simulink model "problematique2"  (Simulink 10.2)
settings: Solver=ode4  StartTime=0.0  StopTime=SIMULPARAM.T_end  FixedStep=SIMULPARAM.Ts  RelTol=1e-3  EnableMultiTasking=on
undefined symbols (not defined in the file): BAT, C_speed, CHAS, Chopper, CYCL, d_current_control, DCBUSCONTROL, dCURRENTCONTROL, ENV, Flux_control, FLUXCONTROL, FLUXSTRATEGY, IM, L, q_current_control, qCURRENTCONTROL, SC, SCCURRENTCONTROL, STRATEGY, TRANS
libraries: simulink x3, cstblocks x1
settings Model: Creator=Huy  LastModifiedBy=mikesimard
settings SolverCC: AlgebraicLoopSolver=LineSearch  AutoInsertRateTranBlk=on
settings DataIOCC: SaveOutput=off  SignalLogging=off  SaveTime=off
settings OptimizationCC: ExpressionDepthLimit=2147483647
settings DebuggingCC: AlgebraicLoopMsg=none  SaveWithDisabledLinksMsg=none  MaxConsecutiveZCsMsg=none  SolverPrmCheckMsg=warning  ModelReferenceDataLoggingMessage=none  ModelReferenceExtraNoncontSigs=none  StateNameClashWarn=warning

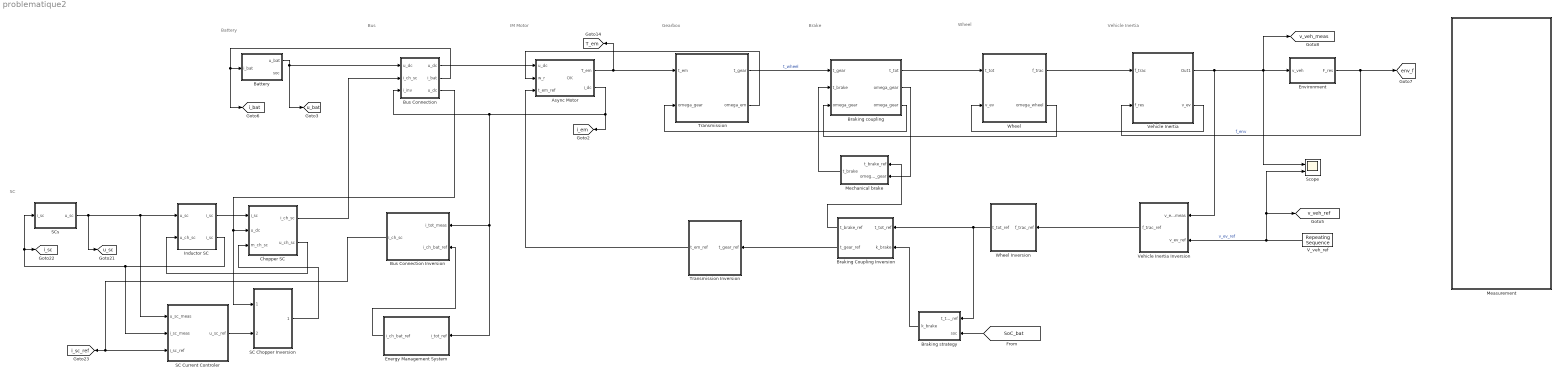
== system problematique2 ==
  note: Battery
  note: Bus
  note: IM Motor
  note: Gearbox
  note: Brake
  note: Wheel
  note: Vehicle Inertia
  note: SC
  note: OK
  Async Motor : Subsystem
  Battery : Subsystem  AncestorBlock=simulink/REM/SE
      mask Display:
      | plot(0,0,100,100, 1.2*[50,57.68,60.77,63.08,64.97,66.58,68,69.26,70.4, 	71.42,72.36,78.28,80,78.28,72.36,71.42,70.4, 	69.26,68,66.58,64.97,63.08,60.77,57.68,50,42.32, 	39.23,36.92,35.03,33.42,32,30.74,29.6,28.58, 	27.64,21.72,20,21.72,27.64,28.58,29.6,30.74,32, 	33.42,35.03,36.92,39.23,42.32,50]-10, 1.2*[20,21,22,23,24,25,26,27,28,29,30,40,50,60,70,71,72, 	73,74,75,76,77,78,79,80,79,78,77,76,75,74,73,72, 	71,70,60,50,40,30,29,28,27,26,25,24,23,22,21,20]-10)
      | disp('ES')
  Braking Coupling Inversion : Subsystem  AncestorBlock=simulink/SMC/Bloc de répartition
      mask Display: plot(0,0,100,100,[20,40,100,80,20],[75,20,20,75,75], [0,20,80,60,0],[85,30,30,85,85])
  Braking coupling : Subsystem  mask(CM){}
      mask Display: plot(0,0,100,100,[35,35,95,95,35],[65,10,10,65,65], [5,5,65,65,5],[90,35,35,90,90])
  Braking strategy : Subsystem  AncestorBlock=simulink/SMC/Inversion EC avec mesure
      mask Display: plot(0,0,100,100,[10,30,90,70,10],[90,10,10,90,90])
  Bus Connection : Subsystem  mask(CM){}
      mask Display: plot(0,0,100,100,[35,35,95,95,35],[65,10,10,65,65], [5,5,65,65,5],[90,35,35,90,90])
  Bus Connection Inversion : Subsystem  AncestorBlock=simulink/SMC/Bloc de répartition
      mask Display: plot(0,0,100,100,[20,40,100,80,20],[75,20,20,75,75], [0,20,80,60,0],[85,30,30,85,85])
  Chopper SC : Subsystem  AncestorBlock=simulink/REM/EC Elec  mask(Hacheur){}
      mask Display: plot(0,0,100,100,[10,10,90,90,10],[90,10,10,90,90])
  Energy Management System : Subsystem  AncestorBlock=simulink/SMC/Inversion EC avec mesure
      mask Display: plot(0,0,100,100,[10,30,90,70,10],[90,10,10,90,90])
  Environment : Subsystem  AncestorBlock=simulink/REM/SE
      mask Display:
      | plot(0,0,100,100, 1.2*[50,57.68,60.77,63.08,64.97,66.58,68,69.26,70.4, 	71.42,72.36,78.28,80,78.28,72.36,71.42,70.4, 	69.26,68,66.58,64.97,63.08,60.77,57.68,50,42.32, 	39.23,36.92,35.03,33.42,32,30.74,29.6,28.58, 	27.64,21.72,20,21.72,27.64,28.58,29.6,30.74,32, 	33.42,35.03,36.92,39.23,42.32,50]-10, 1.2*[20,21,22,23,24,25,26,27,28,29,30,40,50,60,70,71,72, 	73,74,75,76,77,78,79,80,79,78,77,76,75,74,73,72, 	71,70,60,50,40,30,29,28,27,26,25,24,23,22,21,20]-10)
      | disp('MS')
  Inductor SC : Subsystem  AncestorBlock=simulink/REM/EA  mask(CM){}
      mask Display: plot(0,0,100,100,[10,10,90,90,10],[90,10,10,90,90], [10,90],[10,90])
  Measurement : Subsystem
  Mechanical brake : Subsystem  AncestorBlock=simulink/REM/SE
      mask Display:
      | plot(0,0,100,100, 1.2*[50,57.68,60.77,63.08,64.97,66.58,68,69.26,70.4, 	71.42,72.36,78.28,80,78.28,72.36,71.42,70.4, 	69.26,68,66.58,64.97,63.08,60.77,57.68,50,42.32, 	39.23,36.92,35.03,33.42,32,30.74,29.6,28.58, 	27.64,21.72,20,21.72,27.64,28.58,29.6,30.74,32, 	33.42,35.03,36.92,39.23,42.32,50]-10, 1.2*[20,21,22,23,24,25,26,27,28,29,30,40,50,60,70,71,72, 	73,74,75,76,77,78,79,80,79,78,77,76,75,74,73,72, 	71,70,60,50,40,30,29,28,27,26,25,24,23,22,21,20]-10)
      | disp('MS')
  SC Chopper Inversion : Subsystem
      mask Display: plot(0,0,100,100,[10,30,90,70,10],[90,10,10,90,90])
  SC Current Controler : Subsystem
      mask Display: plot(0,0,100,100, [10,30,90,70,10,90],[90,10,10,90,90,10])
  SCs : Subsystem  AncestorBlock=simulink/REM/SE
      mask Display:
      | plot(0,0,100,100, 1.2*[50,57.68,60.77,63.08,64.97,66.58,68,69.26,70.4, 	71.42,72.36,78.28,80,78.28,72.36,71.42,70.4, 	69.26,68,66.58,64.97,63.08,60.77,57.68,50,42.32, 	39.23,36.92,35.03,33.42,32,30.74,29.6,28.58, 	27.64,21.72,20,21.72,27.64,28.58,29.6,30.74,32, 	33.42,35.03,36.92,39.23,42.32,50]-10, 1.2*[20,21,22,23,24,25,26,27,28,29,30,40,50,60,70,71,72, 	73,74,75,76,77,78,79,80,79,78,77,76,75,74,73,72, 	71,70,60,50,40,30,29,28,27,26,25,24,23,22,21,20]-10)
      | disp('ES')
  Scope : Scope  NumInputPorts=2
  Transmission : Subsystem  AncestorBlock=simulink/REM/EA  mask(CM){}
      mask Display: plot(0,0,100,100,[10,10,90,90,10],[90,10,10,90,90])
  Transmission Inversion : Subsystem  AncestorBlock=simulink/SMC/Inversion EC avec mesure
      mask Display: plot(0,0,100,100,[10,30,90,70,10],[90,10,10,90,90])
  V_veh_ref : simulink/Sources/Repeating Sequence  rep_seq_t=CYCL.time  rep_seq_y=CYCL.velocity/1.25
  Vehicle Inertia : Subsystem  AncestorBlock=simulink/REM/EA  mask(CM){}
      mask Display: plot(0,0,100,100,[10,10,90,90,10],[90,10,10,90,90], [10,90],[10,90])
  Vehicle Inertia Inversion : Subsystem  AncestorBlock=simulink/SMC/Asservissement Correcteur IP
      mask Display: plot(0,0,100,100, [10,30,90,70,10,90],[90,10,10,90,90,10])
  Wheel : Subsystem  AncestorBlock=simulink/REM/EA  mask(CM){}
      mask Display: plot(0,0,100,100,[10,10,90,90,10],[90,10,10,90,90])
  Wheel Inversion : Subsystem  AncestorBlock=simulink/SMC/Inversion EC avec mesure
      mask Display: plot(0,0,100,100,[10,30,90,70,10],[90,10,10,90,90])
  tag scope: T_em=global, env_f=global, i_bat=global, i_em=global, i_sc=global, i_sc_ref=global, u_bat=global, u_sc=global, v_veh_meas=global, v_veh_ref=global
  wires:
  Vehicle Inertia/1(Out1) -> Environment/1(v_veh), Scope/1, [v_veh_meas], Vehicle Inertia Inversion/1(v_ev_meas)
  Wheel/1(f_trac) -> Vehicle Inertia/1(f_trac)
  Environment/1(F_res) -> [env_f], Vehicle Inertia/2(f_res)  "f_env"
  Vehicle Inertia/2(v_ev) -> Wheel/2(v_ev)
  V_veh_ref/1 -> Scope/2, [v_veh_ref], Vehicle Inertia Inversion/2(v_ev_ref)  "v_ev_ref"
  Vehicle Inertia Inversion/1(f_trac_ref) -> Wheel Inversion/1(f_trac_ref)
  Transmission/1(t_gear) -> Braking coupling/1(t_gear)  "t_wheel"
  Mechanical brake/1(t_brake) -> Braking coupling/2(t_brake)
  Braking coupling/2(omega_gear) -> Mechanical brake/2(omega_gear)
  Braking Coupling Inversion/2(t_gear_ref) -> Transmission Inversion/1(t_gear_ref)
  Wheel Inversion/1(t_tot_ref) -> Braking strategy/1(t_tot_ref), Braking Coupling Inversion/1(t_tot_ref)
  Braking Coupling Inversion/1(t_brake_ref) -> Mechanical brake/1(t_brake_ref)
  Braking coupling/1(t_tot) -> Wheel/1(t_tot)
  Wheel/2(omega_wheel) -> Braking coupling/3("omega_gear  ")
  Braking coupling/3("omega_gear ") -> Transmission/2(omega_gear)
  Braking strategy/1(k_brake) -> Braking Coupling Inversion/2(k_brake)
  [SoC_bat] -> Braking strategy/2(soc)
  Async Motor/1(T_em) -> Transmission/1(t_em), [T_em]
  Chopper SC/2(u_ch_sc) -> Inductor SC/2(u_ch_sc)
  Inductor SC/1(i_sc) -> Chopper SC/1(i_sc)
  Async Motor/2(i_dc) -> Bus Connection/3(i_inv), Bus Connection Inversion/1(i_tot_meas), Energy Management System/1(i_tot_ref), [i_em]
  Energy Management System/1(i_ch_bat_ref) -> Bus Connection Inversion/2(i_ch_bat_ref)
  SCs/1(u_sc) -> [u_sc], SC Current Controler/1(u_sc_meas), Inductor SC/1(u_sc)
  SC Chopper Inversion/1(m_ch_sc) -> Chopper SC/3(m_ch_sc)
  SC Current Controler/1(u_sc_ref) -> SC Chopper Inversion/2(u_sc_ref)
  Inductor SC/2("i_sc ") -> SC Current Controler/2(i_sc_meas), SCs/1(i_sc), [i_sc]
  Bus Connection Inversion/1(i_ch_sc) -> [i_sc_ref], SC Current Controler/3(i_sc_ref)
  Battery/1(u_bat) -> [u_bat], Bus Connection/1(" u_dc ")
  Bus Connection/3("u_dc ") -> Chopper SC/2(u_dc), SC Chopper Inversion/1(u_dc_meas)
  Transmission/2(omega_em) -> Async Motor/2(w_r)
  Bus Connection/2(i_bat) -> [i_bat], Battery/1(i_bat)
  Bus Connection/1(u_dc) -> Async Motor/1(u_dc)
  Transmission Inversion/1(t_em_ref) -> Async Motor/3(t_em_ref)
  Chopper SC/1(i_ch_sc) -> Bus Connection/2(i_ch_sc)

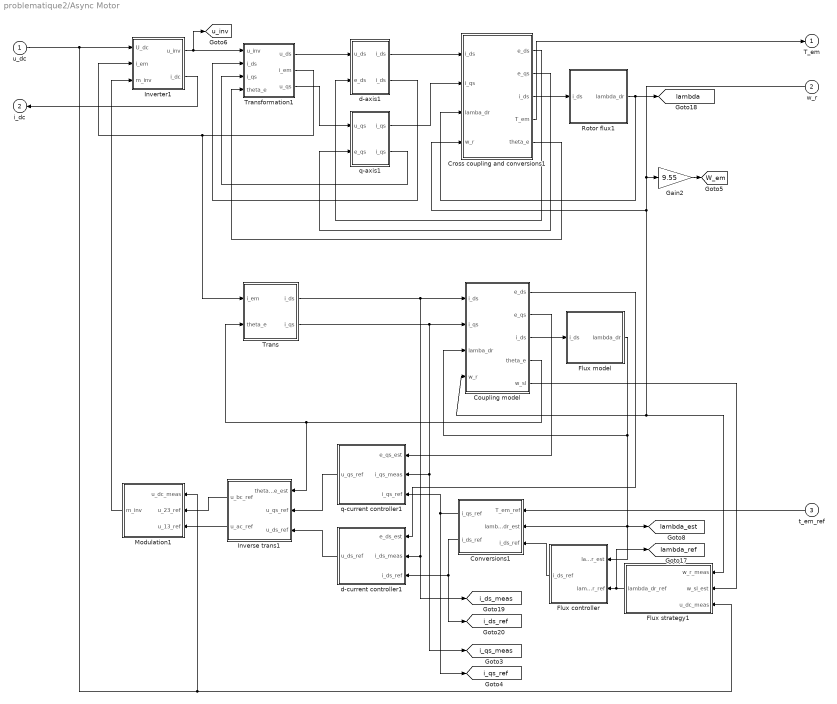
== system problematique2/Async Motor ==
  u_dc : Inport
  w_r : Inport  Port=2
  t_em_ref : Inport  Port=3
  Conversions1 : Subsystem  AncestorBlock=simulink/SMC/Bloc de répartition
      mask Display: plot(0,0,100,100,[20,40,100,80,20],[75,20,20,75,75], [0,20,80,60,0],[85,30,30,85,85])
  Coupling model : Subsystem  AncestorBlock=simulink/REM/EC EM
      mask Display: plot(0,0,100,100, [50,57.68,60.77,63.08,64.97,66.58,68,69.26,70.4, 	71.42,72.36,78.28,80,78.28,72.36,71.42,70.4, 	69.26,68,66.58,64.97,63.08,60.77,57.68,50,42.32, 	39.23,36.92,35.03,33.42,32,30.74,29.6,28.58, 	27.64,21.72,20,21.72,27.64,28.58,29.6,30.74,32, 	33.42,35.03,36.92,39.23,42.32,50], [20,21,22,23,24,25,26,27,28,29,30,40,50,60,70,71,72, 	73,74,75,76,77,78,79,80,79,78,77,76,75,74,73,72, 	71,70,60,50,40,30,29,28,27,26,25,24,23,22,21,20]-15,  [50,57.68,60.77,63.08,64.97,66.58,68,69.26,70.4, 	71.42,72.36,78.28,80,78.28,72.36,71.42,70.4, 	69.26,68,66.58,64.97,63.08,60.77,57.68,50,42.32, 	39.23,36.92,35.03,33.42,32,30.74,29.6,28.58, 	27.64,21.72,20,21.72,27.64,28.58,29.6,30.74,32, 	33.42,35.03,36.92,39.23,42.32,50], [20,21,22,23,24,25,26,27,28,29,30,40,50,60,70,71,72, 	73,74,75,76,77,78,79,80,79,78,77,76,75,74,73,72, 	71,70,60,50,40,30,29,28,27,26,25,24,23,22,21,20]+15)
  Cross coupling and conversions1 : Subsystem  mask(CM){}
      mask Display: plot(0,0,100,100, [50,57.68,60.77,63.08,64.97,66.58,68,69.26,70.4, 	71.42,72.36,78.28,80,78.28,72.36,71.42,70.4, 	69.26,68,66.58,64.97,63.08,60.77,57.68,50,42.32, 	39.23,36.92,35.03,33.42,32,30.74,29.6,28.58, 	27.64,21.72,20,21.72,27.64,28.58,29.6,30.74,32, 	33.42,35.03,36.92,39.23,42.32,50], [20,21,22,23,24,25,26,27,28,29,30,40,50,60,70,71,72, 	73,74,75,76,77,78,79,80,79,78,77,76,75,74,73,72, 	71,70,60,50,40,30,29,28,27,26,25,24,23,22,21,20]-15,  [50,57.68,60.77,63.08,64.97,66.58,68,69.26,70.4, 	71.42,72.36,78.28,80,78.28,72.36,71.42,70.4, 	69.26,68,66.58,64.97,63.08,60.77,57.68,50,42.32, 	39.23,36.92,35.03,33.42,32,30.74,29.6,28.58, 	27.64,21.72,20,21.72,27.64,28.58,29.6,30.74,32, 	33.42,35.03,36.92,39.23,42.32,50], [20,21,22,23,24,25,26,27,28,29,30,40,50,60,70,71,72, 	73,74,75,76,77,78,79,80,79,78,77,76,75,74,73,72, 	71,70,60,50,40,30,29,28,27,26,25,24,23,22,21,20]+15)
  Flux controller : Subsystem  AncestorBlock=simulink/SMC/Asservissement Correcteur IP
      mask Display: plot(0,0,100,100, [10,30,90,70,10,90],[90,10,10,90,90,10])
  Flux model : Subsystem  AncestorBlock=simulink/REM/EA  mask(CM){}
      mask Display: plot(0,0,100,100,[10,10,90,90,10],[90,10,10,90,90], [10,90],[10,90])
  Flux strategy1 : Subsystem  AncestorBlock=simulink/SMC/Inversion EC avec mesure
      mask Display: plot(0,0,100,100,[10,30,90,70,10],[90,10,10,90,90])
  Gain2 : Gain  Gain=9.55
  Inverse trans1 : Subsystem  AncestorBlock=simulink/SMC/Bloc de répartition
      mask Display: plot(0,0,100,100,[20,40,100,80,20],[75,20,20,75,75], [0,20,80,60,0],[85,30,30,85,85])
  Inverter1 : Subsystem  AncestorBlock=simulink/REM/EC Elec  mask(Hacheur){}
      mask Display: plot(0,0,100,100,[10,10,90,90,10],[90,10,10,90,90])
  Modulation1 : Subsystem  AncestorBlock=simulink/SMC/Bloc de répartition
      mask Display: plot(0,0,100,100,[10,30,90,70,10],[90,10,10,90,90])
  Rotor flux1 : Subsystem  AncestorBlock=simulink/REM/EA  mask(CM){}
      mask Display: plot(0,0,100,100,[10,10,90,90,10],[90,10,10,90,90], [10,90],[10,90])
  Trans : Subsystem  mask(CM){}
      mask Display: plot(0,0,100,100,[35,35,95,95,35],[65,10,10,65,65], [5,5,65,65,5],[90,35,35,90,90])
  Transformation1 : Subsystem  mask(CM){}
      mask Display: plot(0,0,100,100,[35,35,95,95,35],[65,10,10,65,65], [5,5,65,65,5],[90,35,35,90,90])
  d-axis1 : Subsystem  AncestorBlock=simulink/REM/EA  mask(CM){}
      mask Display: plot(0,0,100,100,[10,10,90,90,10],[90,10,10,90,90], [10,90],[10,90])
  d-current controller1 : Subsystem  AncestorBlock=simulink/SMC/Asservissement Correcteur IP
      mask Display: plot(0,0,100,100, [10,30,90,70,10,90],[90,10,10,90,90,10])
  q-axis1 : Subsystem  AncestorBlock=simulink/REM/EA  mask(CM){}
      mask Display: plot(0,0,100,100,[10,10,90,90,10],[90,10,10,90,90], [10,90],[10,90])
  q-current controller1 : Subsystem  AncestorBlock=simulink/SMC/Asservissement Correcteur IP
      mask Display: plot(0,0,100,100, [10,30,90,70,10,90],[90,10,10,90,90,10])
  T_em : Outport
  i_dc : Outport  Port=2
  tag scope: W_em=global, i_ds_meas=global, i_ds_ref=global, i_qs_meas=global, i_qs_ref=global, lambda=global, lambda_est=global, lambda_ref=global, u_inv=global
  wires:
  Flux controller/1(i_ds_ref) -> Conversions1/3(i_ds_ref)
  Transformation1/1(u_ds) -> d-axis1/1(u_ds)
  Conversions1/2("i_ds_ref  ") -> d-current controller1/3(i_ds_ref), [i_ds_ref]
  d-axis1/1(i_ds) -> Cross coupling and conversions1/1(i_ds)
  q-axis1/2("i_qs ") -> Transformation1/3(i_qs)
  q-axis1/1(i_qs) -> Cross coupling and conversions1/2(i_qs)
  d-axis1/2("i_ds ") -> Transformation1/2(i_ds)
  Inverse trans1/1(u_bc_ref) -> Modulation1/2(u_23_ref)
  w_r/1 -> Flux strategy1/1(w_r_meas), Coupling model/4(w_r), Cross coupling and conversions1/4(w_r), Gain2/1
  q-current controller1/1(u_qs_ref) -> Inverse trans1/2(u_qs_ref)
  Rotor flux1/1(lambda_dr) -> Cross coupling and conversions1/3(lamba_dr), [lambda]
  Cross coupling and conversions1/4(T_em) -> T_em/1
  u_dc/1 -> Inverter1/1(U_dc), Modulation1/1(u_dc_meas), Flux strategy1/3(u_dc_meas)
  t_em_ref/1 -> Conversions1/1(T_em_ref)
  Inverter1/1(u_inv) -> [u_inv], Transformation1/1(u_inv)
  Coupling model/3("i_ds ") -> Flux model/1(i_ds)
  Gain2/1 -> [W_em]
  Coupling model/4(theta_e) -> Trans/2(theta_e), Inverse trans1/1(theta_e_est)
  Cross coupling and conversions1/3("i_ds ") -> Rotor flux1/1(i_ds)
  Conversions1/1(i_qs_ref) -> [i_qs_ref], q-current controller1/3(i_qs_ref)
  Transformation1/3(u_qs) -> q-axis1/1(u_qs)
  Transformation1/2(i_em) -> Inverter1/2(i_em), Trans/1(i_em)
  Coupling model/2(e_qs) -> q-current controller1/1(e_qs_est)
  Flux strategy1/1(lambda_dr_ref) -> [lambda_ref], Flux controller/2(lambda_dr_ref)
  Trans/1(i_ds) -> Coupling model/1(i_ds), [i_ds_meas], d-current controller1/2(i_ds_meas)
  d-current controller1/1(u_ds_ref) -> Inverse trans1/3(u_ds_ref)
  Cross coupling and conversions1/1(e_ds) -> d-axis1/2(e_ds)
  Coupling model/5(w_sl) -> Flux strategy1/2(w_sl_est)
  Modulation1/1(m_inv) -> Inverter1/3(m_inv)
  Trans/2(i_qs) -> Coupling model/2(i_qs), [i_qs_meas], q-current controller1/2(i_qs_meas)
  Cross coupling and conversions1/2(e_qs) -> q-axis1/2(e_qs)
  Coupling model/1(e_ds) -> d-current controller1/1(e_ds_est)
  Flux model/1(lambda_dr) -> Flux controller/1(lambda_dr_est), [lambda_est], Conversions1/2(lambda_dr_est), Coupling model/3(lamba_dr)
  Cross coupling and conversions1/5(theta_e) -> Transformation1/4(theta_e)
  Inverse trans1/2(u_ac_ref) -> Modulation1/3(u_13_ref)
  Inverter1/2(i_dc) -> i_dc/1

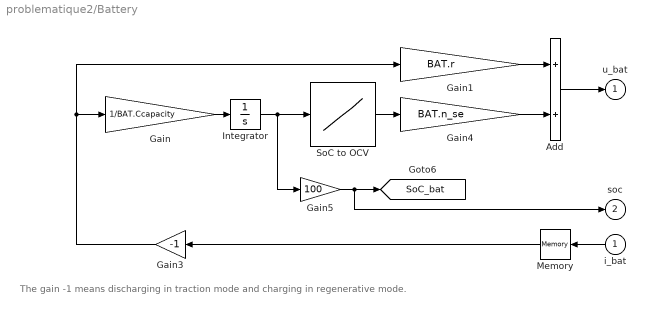
== system problematique2/Battery ==
  note: The gain -1 means discharging in traction mode and charging in regenerative mode.
  i_bat : Inport
  Add : Sum
  Gain : Gain  Gain=1/BAT.Ccapacity
  Gain1 : Gain  Gain=BAT.r
  Gain3 : Gain  Gain=-1
  Gain4 : Gain  Gain=BAT.n_se
  Gain5 : Gain  Gain=100
  Integrator : Integrator  InitialCondition=1
  Memory : Memory
  SoC to OCV : Lookup_n-D  NumberOfTableDimensions=1  BreakpointsForDimension1=0.2:0.1:1  Table=11.4:(12-11.4)/((1-0.2)/0.1):12  RndMeth=Simplest  InputSameDT=on
  u_bat : Outport  InitialOutput=0
  soc : Outport  Port=2  InitialOutput=0
  tag scope: SoC_bat=global
  wires:
  Gain5/1 -> soc/1, [SoC_bat]
  Memory/1 -> Gain3/1
  i_bat/1 -> Memory/1
  Gain/1 -> Integrator/1
  Gain3/1 -> Gain1/1, Gain/1
  SoC to OCV/1 -> Gain4/1
  Integrator/1 -> SoC to OCV/1, Gain5/1
  Gain1/1 -> Add/1
  Add/1 -> u_bat/1
  Gain4/1 -> Add/2

== system problematique2/Braking Coupling Inversion ==
  t_tot_ref : Inport
  k_brake : Inport  Port=2
  Abs : Abs
  Constant : Constant
  Product : Product  RndMeth=Zero
  Product1 : Product  RndMeth=Zero
  Sum : Sum  Inputs=+-
  t_brake_ref : Outport  InitialOutput=0  VectorParamsAs1DForOutWhenUnconnected=off
  t_gear_ref : Outport  Port=2  InitialOutput=0  VectorParamsAs1DForOutWhenUnconnected=off
  wires:
  Product1/1 -> t_gear_ref/1
  Sum/1 -> Product/2
  t_tot_ref/1 -> Product1/1, Product/1
  k_brake/1 -> Product1/2, Sum/2
  Constant/1 -> Sum/1
  Product/1 -> Abs/1
  Abs/1 -> t_brake_ref/1

== system problematique2/Braking coupling ==
  t_gear : Inport
  t_brake : Inport  Port=2
  "omega_gear  " : Inport  Port=3
  Sum : Sum  Inputs=|+-
  t_tot : Outport  InitialOutput=0  VectorParamsAs1DForOutWhenUnconnected=off
  omega_gear : Outport  Port=2  InitialOutput=0  VectorParamsAs1DForOutWhenUnconnected=off
  "omega_gear " : Outport  Port=3  InitialOutput=0  VectorParamsAs1DForOutWhenUnconnected=off
  wires:
  t_gear/1 -> Sum/1
  t_brake/1 -> Sum/2
  Sum/1 -> t_tot/1
  "omega_gear  "/1 -> omega_gear/1, "omega_gear "/1

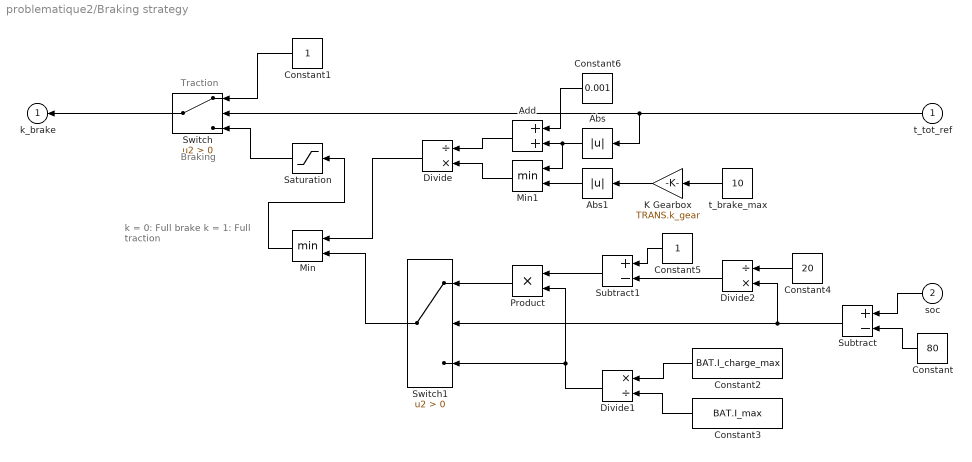
== system problematique2/Braking strategy ==
  note: k = 0: Full brake
      | k = 1: Full traction
  note: Traction
  note: Braking
  t_tot_ref : Inport
  soc : Inport  Port=2
  Abs : Abs
  Abs1 : Abs
  Add : Sum
  Constant : Constant  Value=80
  Constant1 : Constant
  Constant2 : Constant  Value=BAT.I_charge_max
  Constant3 : Constant  Value=BAT.I_max
  Constant4 : Constant  Value=20
  Constant5 : Constant
  Constant6 : Constant  Value=0.001
  Divide : Product  Inputs=/*
  Divide1 : Product  Inputs=*/
  Divide2 : Product  Inputs=/*
  K Gearbox : Gain  Gain=TRANS.k_gear
  Min : MinMax  Inputs=2
  Min1 : MinMax  Inputs=2
  Product : Product
  Saturation : Saturate  UpperLimit=1  LowerLimit=0
  Subtract : Sum  Inputs=+-
  Subtract1 : Sum  Inputs=+-
  Switch : Switch  Criteria=u2 > Threshold
  Switch1 : Switch  Criteria=u2 > Threshold
  t_brake_max : Constant  Value=10
  k_brake : Outport  InitialOutput=0  VectorParamsAs1DForOutWhenUnconnected=off
  wires:
  t_tot_ref/1 -> Abs/1, Switch/2
  Abs/1 -> Add/2, Min1/1
  Abs1/1 -> Min1/2
  Min1/1 -> Divide/2
  Constant/1 -> Subtract/2
  soc/1 -> Subtract/1
  Subtract/1 -> Divide2/2, Switch1/2
  Constant2/1 -> Divide1/1
  Constant3/1 -> Divide1/2
  Divide1/1 -> Switch1/3, Product/2
  Divide2/1 -> Subtract1/2
  Constant5/1 -> Subtract1/1
  Constant4/1 -> Divide2/1
  Product/1 -> Switch1/1
  Subtract1/1 -> Product/1
  t_brake_max/1 -> K Gearbox/1
  K Gearbox/1 -> Abs1/1
  Constant6/1 -> Add/1
  Add/1 -> Divide/1
  Saturation/1 -> Switch/3
  Switch1/1 -> Min/2
  Divide/1 -> Min/1
  Min/1 -> Saturation/1
  Switch/1 -> k_brake/1
  Constant1/1 -> Switch/1

== system problematique2/Bus Connection ==
  " u_dc " : Inport
  i_ch_sc : Inport  Port=2
  i_inv : Inport  Port=3
  Sum : Sum  Inputs=|+-
  u_dc : Outport  InitialOutput=0  VectorParamsAs1DForOutWhenUnconnected=off
  i_bat : Outport  Port=2  InitialOutput=0  VectorParamsAs1DForOutWhenUnconnected=off
  "u_dc " : Outport  Port=3  InitialOutput=0  VectorParamsAs1DForOutWhenUnconnected=off
  wires:
  " u_dc "/1 -> "u_dc "/1, u_dc/1
  Sum/1 -> i_bat/1
  i_inv/1 -> Sum/1
  i_ch_sc/1 -> Sum/2

== system problematique2/Bus Connection Inversion ==
  i_tot_meas : Inport
  i_ch_bat_ref : Inport  Port=2
  Sum : Sum  Inputs=|+-
  i_ch_sc : Outport  InitialOutput=0  VectorParamsAs1DForOutWhenUnconnected=off
  wires:
  i_ch_bat_ref/1 -> Sum/2
  i_tot_meas/1 -> Sum/1
  Sum/1 -> i_ch_sc/1

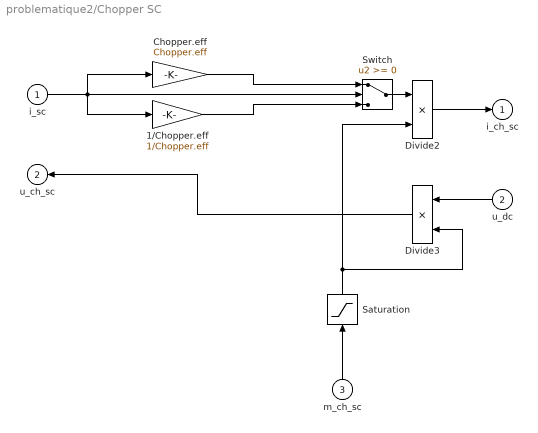
== system problematique2/Chopper SC ==
  i_sc : Inport
  u_dc : Inport  Port=2
  m_ch_sc : Inport  Port=3
  1/Chopper.eff : Gain  Gain=1/Chopper.eff
  Chopper.eff : Gain  Gain=Chopper.eff
  Divide2 : Product  Inputs=**
  Divide3 : Product  Inputs=**
  Saturation : Saturate  UpperLimit=1  LowerLimit=0
  Switch : Switch
  i_ch_sc : Outport  InitialOutput=0  VectorParamsAs1DForOutWhenUnconnected=off
  u_ch_sc : Outport  Port=2  InitialOutput=0  VectorParamsAs1DForOutWhenUnconnected=off
  wires:
  m_ch_sc/1 -> Saturation/1
  1/Chopper.eff/1 -> Switch/3
  Switch/1 -> Divide2/1
  Saturation/1 -> Divide2/2, Divide3/2
  Chopper.eff/1 -> Switch/1
  i_sc/1 -> Chopper.eff/1, 1/Chopper.eff/1, Switch/2
  u_dc/1 -> Divide3/1
  Divide2/1 -> i_ch_sc/1
  Divide3/1 -> u_ch_sc/1

== system problematique2/Energy Management System ==
  i_tot_ref : Inport
  Constant : Constant  Value=STRATEGY.f_c
  Discrete Varying Lowpass : cstblocks/Linear Parameter Varying/Discrete Varying Lowpass  N=1  w0=0  Ts=1
      settings: SourceProductBaseCode=CT
  i_ch_bat_ref : Outport  InitialOutput=0  VectorParamsAs1DForOutWhenUnconnected=off
  wires:
  Constant/1 -> Discrete Varying Lowpass/2
  i_tot_ref/1 -> Discrete Varying Lowpass/1
  Discrete Varying Lowpass/1 -> i_ch_bat_ref/1

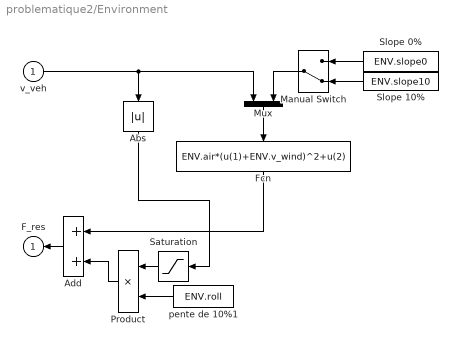
== system problematique2/Environment ==
  v_veh : Inport
  Abs : Abs
  Add : Sum
  Fcn : Fcn  Expr=ENV.air*(u(1)+ENV.v_wind)^2+u(2)
  Manual Switch : ManualSwitch  CurrentSetting=0
  Mux : Mux  Inputs=2
  Product : Product  RndMeth=Zero
  Saturation : Saturate  UpperLimit=1  LowerLimit=0
  Slope 0% : Constant  Value=ENV.slope0
  Slope 10% : Constant  Value=ENV.slope10
  pente de 10%1 : Constant  Value=ENV.roll
  F_res : Outport  InitialOutput=0  VectorParamsAs1DForOutWhenUnconnected=off
  wires:
  Mux/1 -> Fcn/1
  pente de 10%1/1 -> Product/2
  Abs/1 -> Saturation/1
  Fcn/1 -> Add/1
  Product/1 -> Add/2
  Add/1 -> F_res/1
  Slope 0%/1 -> Manual Switch/1
  Slope 10%/1 -> Manual Switch/2
  v_veh/1 -> Mux/1, Abs/1
  Saturation/1 -> Product/1
  Manual Switch/1 -> Mux/2

== system problematique2/Inductor SC ==
  u_sc : Inport
  u_ch_sc : Inport  Port=2
  Inductor SC : TransferFcn  Denominator=[L.SC.L L.SC.r]
  Sum : Sum  Inputs=|+-
  i_sc : Outport  InitialOutput=0  VectorParamsAs1DForOutWhenUnconnected=off
  "i_sc " : Outport  Port=2  InitialOutput=0  VectorParamsAs1DForOutWhenUnconnected=off
  wires:
  u_sc/1 -> Sum/1
  Sum/1 -> Inductor SC/1
  Inductor SC/1 -> i_sc/1, "i_sc "/1
  u_ch_sc/1 -> Sum/2

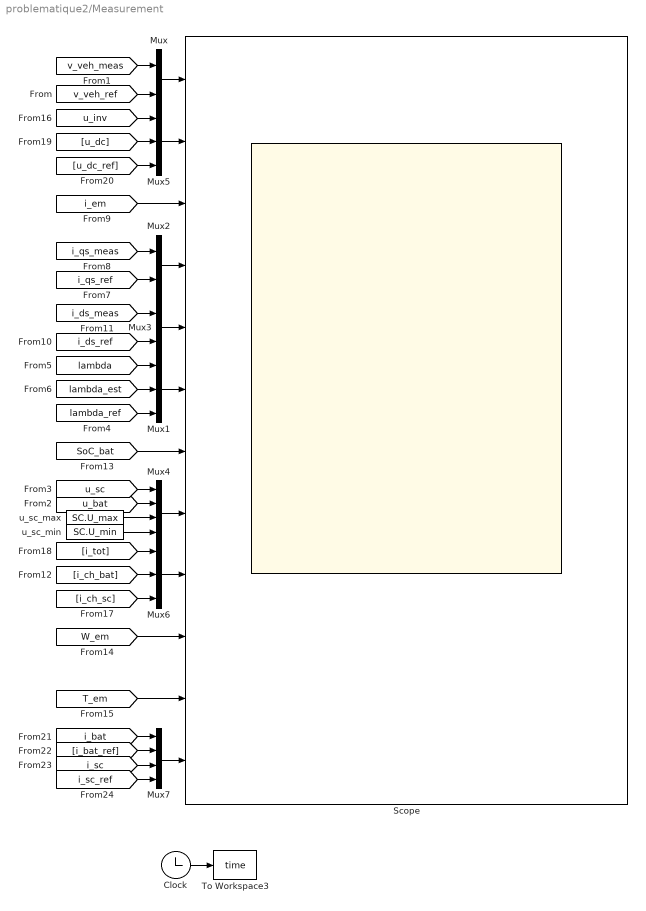
== system problematique2/Measurement ==
  Clock : Clock
      settings: Decimation=10000
  Mux : Mux  Inputs=2
  Mux1 : Mux  Inputs=3
  Mux2 : Mux  Inputs=2
  Mux3 : Mux  Inputs=2
  Mux4 : Mux
  Mux5 : Mux  Inputs=3
  Mux6 : Mux  Inputs=3
  Mux7 : Mux
  Scope : Scope  NumInputPorts=12
  To Workspace3 : ToWorkspace  VariableName=time  SampleTime=-1
      settings: Decimation=SIMULPARAM.Decimation
  u_sc_max : Constant  Value=SC.U_max
  u_sc_min : Constant  Value=SC.U_min
  wires:
  Clock/1 -> To Workspace3/1
  [i_em] -> Scope/3
  [i_ds_meas] -> Mux3/1
  [lambda_ref] -> Mux1/3
  [SoC_bat] -> Scope/7
  [i_qs_meas] -> Mux2/1
  Mux2/1 -> Scope/4
  [i_qs_ref] -> Mux2/2
  [lambda] -> Mux1/1
  [i_ds_ref] -> Mux3/2
  [W_em] -> Scope/10
  [lambda_est] -> Mux1/2
  [v_veh_meas] -> Mux/1
  [v_veh_ref] -> Mux/2
  Mux1/1 -> Scope/6
  Mux/1 -> Scope/1
  [T_em] -> Scope/11
  Mux3/1 -> Scope/5
  [u_dc] -> Mux5/2
  [i_tot] -> Mux6/1
  [u_inv] -> Mux5/1
  u_sc_max/1 -> Mux4/3
  u_sc_min/1 -> Mux4/4
  [u_sc] -> Mux4/1
  [u_bat] -> Mux4/2
  Mux5/1 -> Scope/2
  [i_ch_sc] -> Mux6/3
  Mux4/1 -> Scope/8
  Mux6/1 -> Scope/9
  [u_dc_ref] -> Mux5/3
  [i_ch_bat] -> Mux6/2
  [i_sc] -> Mux7/3
  [i_bat_ref] -> Mux7/2
  [i_sc_ref] -> Mux7/4
  Mux7/1 -> Scope/12
  [i_bat] -> Mux7/1

== system problematique2/Mechanical brake ==
  t_brake_ref : Inport
  omega_gear : Inport  Port=2
  Terminator : Terminator
  t_brake : Outport  InitialOutput=0  VectorParamsAs1DForOutWhenUnconnected=off
  wires:
  t_brake_ref/1 -> t_brake/1
  omega_gear/1 -> Terminator/1

== system problematique2/SC Chopper Inversion ==
  u_dc_meas : Inport
  u_sc_ref : Inport  Port=2
  Divide : Product  Inputs=/*
  Saturation : Saturate  UpperLimit=1  LowerLimit=0
  m_ch_sc : Outport  InitialOutput=0  VectorParamsAs1DForOutWhenUnconnected=off
  wires:
  u_dc_meas/1 -> Divide/1
  Saturation/1 -> m_ch_sc/1
  Divide/1 -> Saturation/1
  u_sc_ref/1 -> Divide/2

== system problematique2/SC Current Controler ==
  u_sc_meas : Inport
  i_sc_meas : Inport  Port=2
  i_sc_ref : Inport  Port=3
  BATCURRENTCONTROL.Ki_pi : Gain  Gain=SCCURRENTCONTROL.Ki_pi
  BATCURRENTCONTROL.Kp_pi : Gain  Gain=SCCURRENTCONTROL.Kp_pi
  Integrator : Integrator
  Sum : Sum  Inputs=|++
  Sum1 : Sum  Inputs=|-+
  Sum3 : Sum  Inputs=|++
  u_sc_ref : Outport  InitialOutput=0
  wires:
  Sum1/1 -> BATCURRENTCONTROL.Ki_pi/1, BATCURRENTCONTROL.Kp_pi/1
  Integrator/1 -> Sum/1
  BATCURRENTCONTROL.Ki_pi/1 -> Integrator/1
  BATCURRENTCONTROL.Kp_pi/1 -> Sum/2
  u_sc_meas/1 -> Sum3/1
  i_sc_ref/1 -> Sum1/2
  i_sc_meas/1 -> Sum1/1
  Sum/1 -> u_sc_ref/1

== system problematique2/SCs ==
  note: The gain -1 means discharging in traction mode and charging in regenerative mode.
  i_sc : Inport
  Add : Sum
  Gain : Gain  Gain=1/SC.C_mod
  Gain1 : Gain  Gain=SC.R_mod
  Gain2 : Gain  Gain=1/SC.n_pa
  Gain3 : Gain  Gain=-1
  Gain4 : Gain  Gain=SC.n_se
  Integrator : Integrator  InitialCondition=SC.U_mod_nom
  u_sc : Outport  InitialOutput=0  VectorParamsAs1DForOutWhenUnconnected=off
  wires:
  Gain2/1 -> Gain3/1
  Gain4/1 -> u_sc/1
  i_sc/1 -> Gain2/1
  Gain1/1 -> Add/1
  Add/1 -> Gain4/1
  Integrator/1 -> Add/2
  Gain/1 -> Integrator/1
  Gain3/1 -> Gain/1, Gain1/1

== system problematique2/Transmission ==
  t_em : Inport
  omega_gear : Inport  Port=2
  1 / ratio1 : Gain  Gain=1/TRANS.k_gear
  gb_eff : Gain  Gain=TRANS.eff
  ratio : Gain  Gain=TRANS.k_gear
  t_gear : Outport  InitialOutput=0
  omega_em : Outport  Port=2  InitialOutput=0
  wires:
  t_em/1 -> ratio/1
  ratio/1 -> gb_eff/1
  gb_eff/1 -> t_gear/1
  omega_gear/1 -> 1 / ratio1/1
  1 / ratio1/1 -> omega_em/1

== system problematique2/Transmission Inversion ==
  t_gear_ref : Inport
  1 / TRAN.k_gear : Gain  Gain=1/TRANS.k_gear
  Braking : Gain  Gain=TRANS.eff
  Switch : Switch
  Traction : Gain  Gain=1/TRANS.eff
  t_em_ref : Outport  InitialOutput=0
  wires:
  1 / TRAN.k_gear/1 -> t_em_ref/1
  t_gear_ref/1 -> Switch/2, Traction/1, Braking/1
  Traction/1 -> Switch/1
  Switch/1 -> 1 / TRAN.k_gear/1
  Braking/1 -> Switch/3

== system problematique2/Vehicle Inertia ==
  f_trac : Inport
  f_res : Inport  Port=2
  1/CHAS.M_veh_tot : Gain  Gain=1/CHAS.M_veh_tot
  Integrator : Integrator
  Sum : Sum  Inputs=|+-
  Out1 : Outport
  v_ev : Outport  Port=2  InitialOutput=0
  wires:
  1/CHAS.M_veh_tot/1 -> Integrator/1
  Integrator/1 -> Out1/1, v_ev/1
  f_trac/1 -> Sum/1
  f_res/1 -> Sum/2
  Sum/1 -> 1/CHAS.M_veh_tot/1

== system problematique2/Vehicle Inertia Inversion ==
  v_ev_meas : Inport
  v_ev_ref : Inport  Port=2
  C_speed.ki : Gain  Gain=C_speed.ki
  C_speed.kp : Gain  Gain=C_speed.kp
  Integrator : Integrator
  Sum : Sum  Inputs=|++
  Sum1 : Sum  Inputs=|-+
  f_trac_ref : Outport  InitialOutput=0
  wires:
  v_ev_ref/1 -> Sum1/2
  v_ev_meas/1 -> Sum1/1
  Sum1/1 -> C_speed.kp/1, C_speed.ki/1
  C_speed.ki/1 -> Integrator/1
  Integrator/1 -> Sum/1
  C_speed.kp/1 -> Sum/2
  Sum/1 -> f_trac_ref/1

== system problematique2/Wheel ==
  t_tot : Inport
  v_ev : Inport  Port=2
  Braking : Gain  Gain=1/TRANS.eff
  Gain : Gain  Gain=TRANS.R_wheel
  Gain1 : Gain  Gain=1/TRANS.R_wheel
  Switch : Switch
  Traction : Gain  Gain=TRANS.eff
  f_trac : Outport  InitialOutput=0
  omega_wheel : Outport  Port=2  InitialOutput=0
  wires:
  Gain1/1 -> f_trac/1
  v_ev/1 -> Gain/1
  Braking/1 -> Switch/3
  Switch/1 -> Gain1/1
  Gain/1 -> omega_wheel/1
  Traction/1 -> Switch/1
  t_tot/1 -> Traction/1, Switch/2, Braking/1

== system problematique2/Wheel Inversion ==
  f_trac_ref : Inport
  1/TRANS.r_wheel : Gain  Gain=TRANS.R_wheel
  t_tot_ref : Outport  InitialOutput=0
  wires:
  f_trac_ref/1 -> 1/TRANS.r_wheel/1
  1/TRANS.r_wheel/1 -> t_tot_ref/1

== system problematique2/Async Motor/Conversions1 ==
  T_em_ref : Inport
  lambda_dr_est : Inport  Port=2
  i_ds_ref : Inport  Port=3
  Constant : Constant  Value=1e-6
  Mux1 : Mux  Inputs=2
  Sum : Sum  Inputs=|++
  i_qs_ref cal : Fcn  Expr=u(1)/((3/2)*IM.pp*(IM.Lm/IM.Lr)*u(2))
  i_qs_ref : Outport  InitialOutput=0  VectorParamsAs1DForOutWhenUnconnected=off
  "i_ds_ref  " : Outport  Port=2  InitialOutput=0  VectorParamsAs1DForOutWhenUnconnected=off
  wires:
  Mux1/1 -> i_qs_ref cal/1
  i_qs_ref cal/1 -> i_qs_ref/1
  i_ds_ref/1 -> "i_ds_ref  "/1
  T_em_ref/1 -> Mux1/1
  lambda_dr_est/1 -> Sum/1
  Sum/1 -> Mux1/2
  Constant/1 -> Sum/2

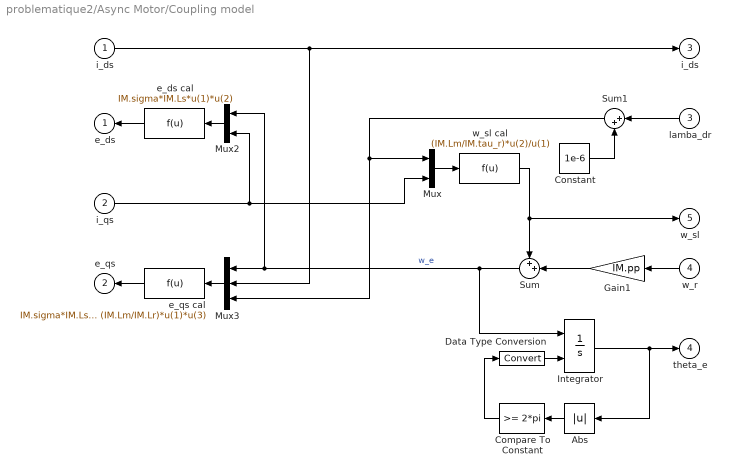
== system problematique2/Async Motor/Coupling model ==
  i_ds : Inport
  i_qs : Inport  Port=2
  lamba_dr : Inport  Port=3
  w_r : Inport  Port=4
  Abs : Abs
  Compare To Constant : simulink/Logic and Bit Operations/Compare To Constant  relop=>=  const=2*pi  OutDataTypeStr=boolean  ZeroCross=off
  Constant : Constant  Value=1e-6
  Data Type Conversion : DataTypeConversion
  Gain1 : Gain  Gain=IM.pp
  Integrator : Integrator  ExternalReset=level
  Mux : Mux  Inputs=2
  Mux2 : Mux  Inputs=2
  Mux3 : Mux  Inputs=3
  Sum : Sum  Inputs=++|
  Sum1 : Sum  Inputs=|++
  e_ds cal : Fcn  Expr=IM.sigma*IM.Ls*u(1)*u(2)
  e_qs cal : Fcn  Expr=IM.sigma*IM.Ls*u(1)*u(2) + (IM.Lm/IM.Lr)*u(1)*u(3)
  w_sl cal : Fcn  Expr=(IM.Lm/IM.tau_r)*u(2)/u(1)
  e_ds : Outport  InitialOutput=0  VectorParamsAs1DForOutWhenUnconnected=off
  e_qs : Outport  Port=2  InitialOutput=0  VectorParamsAs1DForOutWhenUnconnected=off
  "i_ds " : Outport  Port=3  InitialOutput=0  VectorParamsAs1DForOutWhenUnconnected=off
  theta_e : Outport  Port=4  InitialOutput=0  VectorParamsAs1DForOutWhenUnconnected=off
  w_sl : Outport  Port=5  InitialOutput=0  VectorParamsAs1DForOutWhenUnconnected=off
  wires:
  i_ds/1 -> "i_ds "/1, Mux3/2
  Mux/1 -> w_sl cal/1
  i_qs/1 -> Mux2/2, Mux/2
  w_r/1 -> Gain1/1
  w_sl cal/1 -> w_sl/1, Sum/1
  Mux2/1 -> e_ds cal/1
  e_ds cal/1 -> e_ds/1
  Sum/1 -> Integrator/1, Mux2/1, Mux3/1  "w_e"
  Mux3/1 -> e_qs cal/1
  e_qs cal/1 -> e_qs/1
  Sum1/1 -> Mux/1, Mux3/3
  lamba_dr/1 -> Sum1/1
  Constant/1 -> Sum1/2
  Integrator/1 -> theta_e/1, Abs/1
  Abs/1 -> Compare To Constant/1
  Compare To Constant/1 -> Data Type Conversion/1
  Data Type Conversion/1 -> Integrator/2
  Gain1/1 -> Sum/2

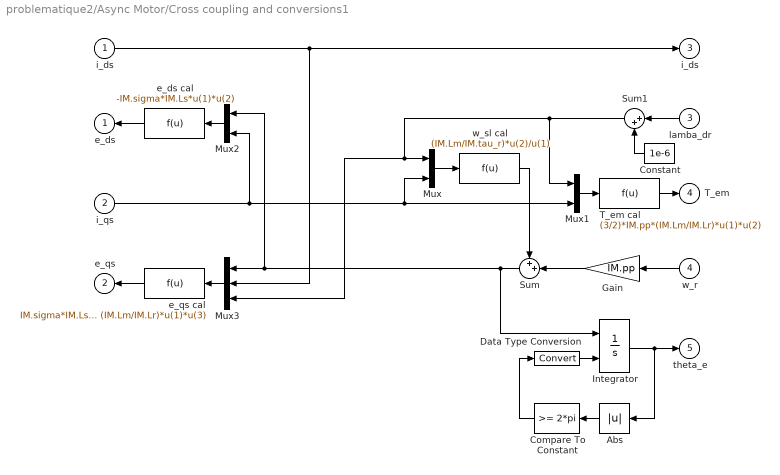
== system problematique2/Async Motor/Cross coupling and conversions1 ==
  i_ds : Inport
  i_qs : Inport  Port=2
  lamba_dr : Inport  Port=3
  w_r : Inport  Port=4
  Abs : Abs
  Compare To Constant : simulink/Logic and Bit Operations/Compare To Constant  relop=>=  const=2*pi  OutDataTypeStr=boolean  ZeroCross=off
  Constant : Constant  Value=1e-6
  Data Type Conversion : DataTypeConversion
  Gain : Gain  Gain=IM.pp
  Integrator : Integrator  ExternalReset=level
  Mux : Mux  Inputs=2
  Mux1 : Mux  Inputs=2
  Mux2 : Mux  Inputs=2
  Mux3 : Mux  Inputs=3
  Sum : Sum  Inputs=++|
  Sum1 : Sum  Inputs=|++
  T_em cal : Fcn  Expr=(3/2)*IM.pp*(IM.Lm/IM.Lr)*u(1)*u(2)
  e_ds cal : Fcn  Expr=-IM.sigma*IM.Ls*u(1)*u(2)
  e_qs cal : Fcn  Expr=IM.sigma*IM.Ls*u(1)*u(2) + (IM.Lm/IM.Lr)*u(1)*u(3)
  w_sl cal : Fcn  Expr=(IM.Lm/IM.tau_r)*u(2)/u(1)
  e_ds : Outport  InitialOutput=0  VectorParamsAs1DForOutWhenUnconnected=off
  e_qs : Outport  Port=2  InitialOutput=0  VectorParamsAs1DForOutWhenUnconnected=off
  "i_ds " : Outport  Port=3  InitialOutput=0  VectorParamsAs1DForOutWhenUnconnected=off
  T_em : Outport  Port=4  InitialOutput=0  VectorParamsAs1DForOutWhenUnconnected=off
  theta_e : Outport  Port=5  InitialOutput=0  VectorParamsAs1DForOutWhenUnconnected=off
  wires:
  Mux3/1 -> e_qs cal/1
  Integrator/1 -> theta_e/1, Abs/1
  Compare To Constant/1 -> Data Type Conversion/1
  lamba_dr/1 -> Sum1/1
  e_qs cal/1 -> e_qs/1
  Gain/1 -> Sum/2
  Sum1/1 -> Mux1/1, Mux/1, Mux3/3
  i_qs/1 -> Mux/2, Mux1/2, Mux2/2
  Data Type Conversion/1 -> Integrator/2
  Mux2/1 -> e_ds cal/1
  T_em cal/1 -> T_em/1
  Mux1/1 -> T_em cal/1
  e_ds cal/1 -> e_ds/1
  w_r/1 -> Gain/1
  Abs/1 -> Compare To Constant/1
  Constant/1 -> Sum1/2
  Sum/1 -> Mux2/1, Mux3/1, Integrator/1
  i_ds/1 -> "i_ds "/1, Mux3/2
  Mux/1 -> w_sl cal/1
  w_sl cal/1 -> Sum/1

== system problematique2/Async Motor/Flux controller ==
  lambda_dr_est : Inport
  lambda_dr_ref : Inport  Port=2
  Constant : Constant  Value=Flux_control
  IP controller : Subsystem
  Multiport Switch : MultiPortSwitch  Inputs=2
  PI controller : Subsystem
  i_ds_ref : Outport  InitialOutput=0  VectorParamsAs1DForOutWhenUnconnected=off
  wires:
  lambda_dr_est/1 -> IP controller/1(lambda_dr_est), PI controller/1(lambda_dr_est)
  lambda_dr_ref/1 -> IP controller/2(lambda_dr_ref), PI controller/2(lambda_dr_ref)
  Constant/1 -> Multiport Switch/1
  IP controller/1(i_ds_ref) -> Multiport Switch/3
  PI controller/1(i_ds_ref) -> Multiport Switch/2
  Multiport Switch/1 -> i_ds_ref/1

== system problematique2/Async Motor/Flux model ==
  i_ds : Inport
  Magnetization : TransferFcn  Numerator=[IM.Lm]  Denominator=[IM.tau_r 1]
  lambda_dr : Outport  InitialOutput=0  VectorParamsAs1DForOutWhenUnconnected=off
  wires:
  i_ds/1 -> Magnetization/1
  Magnetization/1 -> lambda_dr/1

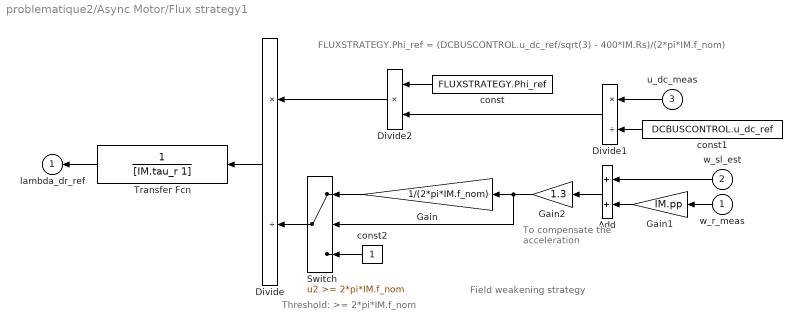
== system problematique2/Async Motor/Flux strategy1 ==
  note: Field weakening strategy
  note: To compensate
      | the acceleration
  note: FLUXSTRATEGY.Phi_ref = (DCBUSCONTROL.u_dc_ref/sqrt(3) - 400*IM.Rs)/(2*pi*IM.f_nom)
  note: Threshold: >= 2*pi*IM.f_nom
  w_r_meas : Inport
  w_sl_est : Inport  Port=2
  u_dc_meas : Inport  Port=3
  Add : Sum
  Divide : Product  Inputs=*/
  Divide1 : Product  Inputs=*/
  Divide2 : Product  Inputs=**
  Gain : Gain  Gain=1/(2*pi*IM.f_nom)
  Gain1 : Gain  Gain=IM.pp
  Gain2 : Gain  Gain=1.3
  Switch : Switch  Threshold=2*pi*IM.f_nom
  Transfer Fcn : TransferFcn  Denominator=[IM.tau_r 1]
  const : Constant  Value=FLUXSTRATEGY.Phi_ref
  const1 : Constant  Value=DCBUSCONTROL.u_dc_ref
  const2 : Constant
  lambda_dr_ref : Outport  InitialOutput=0  VectorParamsAs1DForOutWhenUnconnected=off
  wires:
  w_r_meas/1 -> Gain1/1
  Add/1 -> Gain2/1
  Gain1/1 -> Add/2
  w_sl_est/1 -> Add/1
  const1/1 -> Divide1/2
  u_dc_meas/1 -> Divide1/1
  Divide1/1 -> Divide2/2
  const/1 -> Divide2/1
  Divide2/1 -> Divide/1
  Gain/1 -> Switch/1
  Switch/1 -> Divide/2
  const2/1 -> Switch/3
  Gain2/1 -> Switch/2, Gain/1
  Divide/1 -> Transfer Fcn/1
  Transfer Fcn/1 -> lambda_dr_ref/1

== system problematique2/Async Motor/Inverse trans1 ==
  theta_e_est : Inport
  u_qs_ref : Inport  Port=2
  u_ds_ref : Inport  Port=3
  dq2line voltage : Subsystem
  u_bc_ref : Outport  InitialOutput=0  VectorParamsAs1DForOutWhenUnconnected=off
  u_ac_ref : Outport  Port=2  InitialOutput=0  VectorParamsAs1DForOutWhenUnconnected=off
  wires:
  dq2line voltage/2(2) -> u_bc_ref/1
  dq2line voltage/1(1) -> u_ac_ref/1
  theta_e_est/1 -> dq2line voltage/3(theta)
  u_qs_ref/1 -> dq2line voltage/2(q)
  u_ds_ref/1 -> dq2line voltage/1(d)

== system problematique2/Async Motor/Inverter1 ==
  U_dc : Inport
  i_em : Inport  Port=2
  m_inv : Inport  Port=3
  Divide : Product  Inputs=**
  Divide1 : Product  Inputs=**
  Saturation : Saturate  UpperLimit=1  LowerLimit=-1
  Sum of Elements : Sum  Inputs=+
  u_inv : Outport  InitialOutput=0  VectorParamsAs1DForOutWhenUnconnected=off
  i_dc : Outport  Port=2  InitialOutput=0  VectorParamsAs1DForOutWhenUnconnected=off
  wires:
  i_em/1 -> Divide1/1
  m_inv/1 -> Saturation/1
  Divide/1 -> u_inv/1
  U_dc/1 -> Divide/1
  Sum of Elements/1 -> i_dc/1
  Divide1/1 -> Sum of Elements/1
  Saturation/1 -> Divide/2, Divide1/2

== system problematique2/Async Motor/Modulation1 ==
  u_dc_meas : Inport
  u_23_ref : Inport  Port=2
  u_13_ref : Inport  Port=3
  Divide : Product  Inputs=/*
  Mux : Mux  Inputs=2
  Saturation : Saturate  UpperLimit=1  LowerLimit=-1
  m_inv : Outport  InitialOutput=0  VectorParamsAs1DForOutWhenUnconnected=off
  wires:
  u_dc_meas/1 -> Divide/1
  Mux/1 -> Divide/2
  u_23_ref/1 -> Mux/2
  u_13_ref/1 -> Mux/1
  Divide/1 -> Saturation/1
  Saturation/1 -> m_inv/1

== system problematique2/Async Motor/Rotor flux1 ==
  i_ds : Inport
  Magnetization : TransferFcn  Numerator=[IM.Lm]  Denominator=[IM.tau_r 1]
  lambda_dr : Outport  InitialOutput=0  VectorParamsAs1DForOutWhenUnconnected=off
  wires:
  i_ds/1 -> Magnetization/1
  Magnetization/1 -> lambda_dr/1

== system problematique2/Async Motor/Trans ==
  i_em : Inport
  theta_e : Inport  Port=2
  Demux : Demux  Outputs=2
  current line2dq : Subsystem
  i_ds : Outport  InitialOutput=0  VectorParamsAs1DForOutWhenUnconnected=off
  i_qs : Outport  Port=2  InitialOutput=0  VectorParamsAs1DForOutWhenUnconnected=off
  wires:
  i_em/1 -> Demux/1
  Demux/1 -> current line2dq/1(1)
  Demux/2 -> current line2dq/2(2)
  current line2dq/1(d) -> i_ds/1
  current line2dq/2(q) -> i_qs/1
  theta_e/1 -> current line2dq/3(theta)

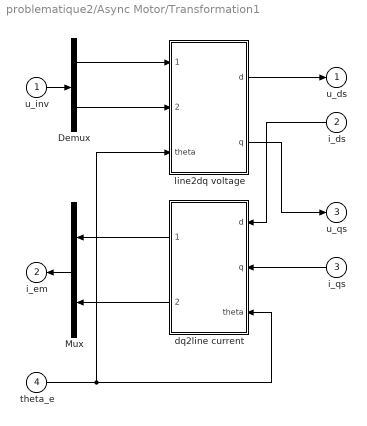
== system problematique2/Async Motor/Transformation1 ==
  u_inv : Inport
  i_ds : Inport  Port=2
  i_qs : Inport  Port=3
  theta_e : Inport  Port=4
  Demux : Demux  Outputs=2
  Mux : Mux  Inputs=2
  dq2line current : Subsystem
  line2dq voltage : Subsystem
  u_ds : Outport  InitialOutput=0  VectorParamsAs1DForOutWhenUnconnected=off
  i_em : Outport  Port=2  InitialOutput=0  VectorParamsAs1DForOutWhenUnconnected=off
  u_qs : Outport  Port=3  InitialOutput=0  VectorParamsAs1DForOutWhenUnconnected=off
  wires:
  line2dq voltage/1(d) -> u_ds/1
  line2dq voltage/2(q) -> u_qs/1
  i_ds/1 -> dq2line current/1(d)
  i_qs/1 -> dq2line current/2(q)
  u_inv/1 -> Demux/1
  Mux/1 -> i_em/1
  Demux/1 -> line2dq voltage/1(1)
  Demux/2 -> line2dq voltage/2(2)
  theta_e/1 -> line2dq voltage/3(theta), dq2line current/3(theta)
  dq2line current/1(1) -> Mux/1
  dq2line current/2(2) -> Mux/2

== system problematique2/Async Motor/d-axis1 ==
  u_ds : Inport
  e_ds : Inport  Port=2
  Sum : Sum  Inputs=|+-
  d-axis : TransferFcn  Denominator=[IM.sigma*IM.Ls IM.Rs]
  i_ds : Outport  InitialOutput=0  VectorParamsAs1DForOutWhenUnconnected=off
  "i_ds " : Outport  Port=2  InitialOutput=0  VectorParamsAs1DForOutWhenUnconnected=off
  wires:
  e_ds/1 -> Sum/2
  d-axis/1 -> "i_ds "/1, i_ds/1
  Sum/1 -> d-axis/1
  u_ds/1 -> Sum/1

== system problematique2/Async Motor/d-current controller1 ==
  e_ds_est : Inport
  i_ds_meas : Inport  Port=2
  i_ds_ref : Inport  Port=3
  Constant : Constant  Value=d_current_control
  IP controller : Subsystem
  Multiport Switch : MultiPortSwitch  Inputs=2
  PI controller : Subsystem
  Sum2 : Sum  Inputs=++|
  u_ds_ref : Outport  InitialOutput=0  VectorParamsAs1DForOutWhenUnconnected=off
  wires:
  e_ds_est/1 -> Sum2/1
  Sum2/1 -> u_ds_ref/1
  Constant/1 -> Multiport Switch/1
  IP controller/1(u_ds_arm) -> Multiport Switch/3
  PI controller/1(u_ds_arm) -> Multiport Switch/2
  i_ds_meas/1 -> IP controller/1(i_ds_meas), PI controller/1(i_ds_meas)
  i_ds_ref/1 -> IP controller/2(i_ds_ref), PI controller/2(i_ds_ref)
  Multiport Switch/1 -> Sum2/2

== system problematique2/Async Motor/q-axis1 ==
  u_qs : Inport
  e_qs : Inport  Port=2
  Sum : Sum  Inputs=|+-
  q-axis : TransferFcn  Denominator=[IM.sigma*IM.Ls IM.Rs]
  i_qs : Outport  InitialOutput=0  VectorParamsAs1DForOutWhenUnconnected=off
  "i_qs " : Outport  Port=2  InitialOutput=0  VectorParamsAs1DForOutWhenUnconnected=off
  wires:
  u_qs/1 -> Sum/1
  Sum/1 -> q-axis/1
  q-axis/1 -> i_qs/1, "i_qs "/1
  e_qs/1 -> Sum/2

== system problematique2/Async Motor/q-current controller1 ==
  e_qs_est : Inport
  i_qs_meas : Inport  Port=2
  i_qs_ref : Inport  Port=3
  Constant : Constant  Value=q_current_control
  IP controller : Subsystem
  Multiport Switch : MultiPortSwitch  Inputs=2
  PI controller : Subsystem
  Sum2 : Sum  Inputs=++|
  u_qs_ref : Outport  InitialOutput=0  VectorParamsAs1DForOutWhenUnconnected=off
  wires:
  e_qs_est/1 -> Sum2/1
  Sum2/1 -> u_qs_ref/1
  Constant/1 -> Multiport Switch/1
  IP controller/1(u_qs_arm) -> Multiport Switch/3
  PI controller/1(u_qs_arm) -> Multiport Switch/2
  i_qs_meas/1 -> IP controller/1(i_qs_meas), PI controller/1(i_qs_meas)
  i_qs_ref/1 -> IP controller/2(i_qs_ref), PI controller/2(i_qs_ref)
  Multiport Switch/1 -> Sum2/2

== system problematique2/Async Motor/Flux controller/IP controller ==
  lambda_dr_est : Inport
  lambda_dr_ref : Inport  Port=2
  Gain : Gain  Gain=FLUXCONTROL.Kp_ip
  Gain1 : Gain  Gain=FLUXCONTROL.Ki_ip
  Integrator : Integrator
  Sum : Sum  Inputs=+-
  Sum1 : Sum  Inputs=-+
  i_ds_ref : Outport  VectorParamsAs1DForOutWhenUnconnected=off
  wires:
  Sum/1 -> i_ds_ref/1
  Sum1/1 -> Gain1/1
  lambda_dr_est/1 -> Gain/1, Sum1/1
  lambda_dr_ref/1 -> Sum1/2
  Gain1/1 -> Integrator/1
  Integrator/1 -> Sum/1
  Gain/1 -> Sum/2

== system problematique2/Async Motor/Flux controller/PI controller ==
  lambda_dr_est : Inport
  lambda_dr_ref : Inport  Port=2
  Gain : Gain  Gain=FLUXCONTROL.Kp_pi
  Gain1 : Gain  Gain=FLUXCONTROL.Ki_pi
  Integrator : Integrator
  Sum : Sum
  Sum1 : Sum  Inputs=-+
  i_ds_ref : Outport  VectorParamsAs1DForOutWhenUnconnected=off
  wires:
  Gain1/1 -> Integrator/1
  lambda_dr_est/1 -> Sum1/1
  Gain/1 -> Sum/1
  Sum1/1 -> Gain1/1, Gain/1
  Integrator/1 -> Sum/2
  Sum/1 -> i_ds_ref/1
  lambda_dr_ref/1 -> Sum1/2

== system problematique2/Async Motor/Inverse trans1/dq2line voltage ==
  d : Inport
  q : Inport  Port=2
  theta : Inport  Port=3
  Add2 : Sum  Inputs=+-
  Add3 : Sum  Inputs=+-
  albe2abc : Subsystem
  dq2albe : Subsystem
  1 : Outport  VectorParamsAs1DForOutWhenUnconnected=off
  2 : Outport  Port=2  VectorParamsAs1DForOutWhenUnconnected=off
  wires:
  dq2albe/1(alpha) -> albe2abc/1(alpha)
  dq2albe/2(beta) -> albe2abc/2(beta)
  albe2abc/2(b) -> Add3/1
  albe2abc/1(a) -> Add2/1
  albe2abc/3(c) -> Add3/2, Add2/2
  Add2/1 -> 1/1
  Add3/1 -> 2/1
  d/1 -> dq2albe/1(d)
  q/1 -> dq2albe/2(q)
  theta/1 -> dq2albe/3(theta)

== system problematique2/Async Motor/Trans/current line2dq ==
  1 : Inport
  2 : Inport  Port=2
  theta : Inport  Port=3
  Add : Sum  Inputs=--
  abc2albe : Subsystem
  albe2dq : Subsystem
  d : Outport  VectorParamsAs1DForOutWhenUnconnected=off
  q : Outport  Port=2  VectorParamsAs1DForOutWhenUnconnected=off
  wires:
  albe2dq/1(d) -> d/1
  albe2dq/2(q) -> q/1
  abc2albe/1(alpha) -> albe2dq/1(alpha)
  abc2albe/2(beta) -> albe2dq/2(beta)
  theta/1 -> albe2dq/3(theta)
  Add/1 -> abc2albe/3(c)
  2/1 -> abc2albe/2(b), Add/2
  1/1 -> abc2albe/1(a), Add/1

== system problematique2/Async Motor/Transformation1/dq2line current ==
  d : Inport
  q : Inport  Port=2
  theta : Inport  Port=3
  Terminator : Terminator
  albe2abc : Subsystem
  dq2albe : Subsystem
  1 : Outport  VectorParamsAs1DForOutWhenUnconnected=off
  2 : Outport  Port=2  VectorParamsAs1DForOutWhenUnconnected=off
  wires:
  dq2albe/1(alpha) -> albe2abc/1(alpha)
  dq2albe/2(beta) -> albe2abc/2(beta)
  albe2abc/1(a) -> 1/1
  albe2abc/2(b) -> 2/1
  d/1 -> dq2albe/1(d)
  q/1 -> dq2albe/2(q)
  theta/1 -> dq2albe/3(theta)
  albe2abc/3(c) -> Terminator/1

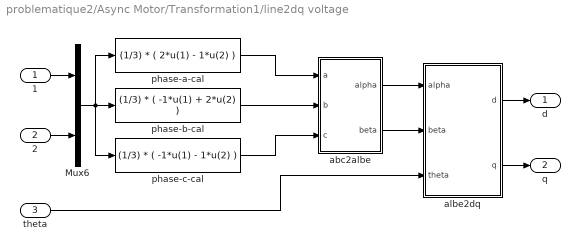
== system problematique2/Async Motor/Transformation1/line2dq voltage ==
  1 : Inport
  2 : Inport  Port=2
  theta : Inport  Port=3
  Mux6 : Mux  Inputs=2
  abc2albe : Subsystem
  albe2dq : Subsystem
  phase-a-cal : Fcn  Expr=(1/3) * ( 2*u(1) - 1*u(2) )
  phase-b-cal : Fcn  Expr=(1/3) * ( -1*u(1) + 2*u(2) )
  phase-c-cal : Fcn  Expr=(1/3) * ( -1*u(1) - 1*u(2) )
  d : Outport  VectorParamsAs1DForOutWhenUnconnected=off
  q : Outport  Port=2  VectorParamsAs1DForOutWhenUnconnected=off
  wires:
  albe2dq/1(d) -> d/1
  albe2dq/2(q) -> q/1
  1/1 -> Mux6/1
  2/1 -> Mux6/2
  abc2albe/1(alpha) -> albe2dq/1(alpha)
  abc2albe/2(beta) -> albe2dq/2(beta)
  phase-b-cal/1 -> abc2albe/2(b)
  phase-a-cal/1 -> abc2albe/1(a)
  phase-c-cal/1 -> abc2albe/3(c)
  Mux6/1 -> phase-b-cal/1, phase-c-cal/1, phase-a-cal/1
  theta/1 -> albe2dq/3(theta)

== system problematique2/Async Motor/d-current controller1/IP controller ==
  i_ds_meas : Inport
  i_ds_ref : Inport  Port=2
  Gain : Gain  Gain=dCURRENTCONTROL.Kp_ip
  Gain1 : Gain  Gain=dCURRENTCONTROL.Ki_ip
  Integrator : Integrator
  Sum : Sum  Inputs=+-
  Sum1 : Sum  Inputs=-+
  u_ds_arm : Outport  VectorParamsAs1DForOutWhenUnconnected=off
  wires:
  Gain1/1 -> Integrator/1
  i_ds_ref/1 -> Sum1/2
  i_ds_meas/1 -> Gain/1, Sum1/1
  Sum1/1 -> Gain1/1
  Sum/1 -> u_ds_arm/1
  Integrator/1 -> Sum/1
  Gain/1 -> Sum/2

== system problematique2/Async Motor/d-current controller1/PI controller ==
  i_ds_meas : Inport
  i_ds_ref : Inport  Port=2
  Gain : Gain  Gain=dCURRENTCONTROL.Kp_pi
  Gain1 : Gain  Gain=dCURRENTCONTROL.Ki_pi
  Integrator : Integrator
  Sum : Sum
  Sum1 : Sum  Inputs=-+
  u_ds_arm : Outport  VectorParamsAs1DForOutWhenUnconnected=off
  wires:
  Gain/1 -> Sum/1
  Sum/1 -> u_ds_arm/1
  Sum1/1 -> Gain1/1, Gain/1
  i_ds_meas/1 -> Sum1/1
  Integrator/1 -> Sum/2
  i_ds_ref/1 -> Sum1/2
  Gain1/1 -> Integrator/1

== system problematique2/Async Motor/q-current controller1/IP controller ==
  i_qs_meas : Inport
  i_qs_ref : Inport  Port=2
  Gain : Gain  Gain=qCURRENTCONTROL.Kp_ip
  Gain1 : Gain  Gain=qCURRENTCONTROL.Ki_ip
  Integrator : Integrator
  Sum : Sum  Inputs=+-
  Sum1 : Sum  Inputs=-+
  u_qs_arm : Outport  VectorParamsAs1DForOutWhenUnconnected=off
  wires:
  Gain1/1 -> Integrator/1
  i_qs_ref/1 -> Sum1/2
  i_qs_meas/1 -> Gain/1, Sum1/1
  Sum1/1 -> Gain1/1
  Sum/1 -> u_qs_arm/1
  Integrator/1 -> Sum/1
  Gain/1 -> Sum/2

== system problematique2/Async Motor/q-current controller1/PI controller ==
  i_qs_meas : Inport
  i_qs_ref : Inport  Port=2
  Gain : Gain  Gain=qCURRENTCONTROL.Kp_pi
  Gain1 : Gain  Gain=qCURRENTCONTROL.Ki_pi
  Integrator : Integrator
  Sum : Sum
  Sum1 : Sum  Inputs=-+
  u_qs_arm : Outport  VectorParamsAs1DForOutWhenUnconnected=off
  wires:
  Gain/1 -> Sum/1
  Sum/1 -> u_qs_arm/1
  Sum1/1 -> Gain1/1, Gain/1
  i_qs_meas/1 -> Sum1/1
  Integrator/1 -> Sum/2
  i_qs_ref/1 -> Sum1/2
  Gain1/1 -> Integrator/1

== system problematique2/Async Motor/Inverse trans1/dq2line voltage/albe2abc ==
  alpha : Inport
  beta : Inport  Port=2
  Mux : Mux  Inputs=2
  a-cal : Fcn  Expr=u(1)
  b-cal : Fcn  Expr=(-u(1) + sqrt(3)*u(2))/2
  c-cal : Fcn  Expr=(-u(1) - sqrt(3)*u(2))/2
  a : Outport  VectorParamsAs1DForOutWhenUnconnected=off
  b : Outport  Port=2  VectorParamsAs1DForOutWhenUnconnected=off
  c : Outport  Port=3  VectorParamsAs1DForOutWhenUnconnected=off
  wires:
  alpha/1 -> Mux/1
  beta/1 -> Mux/2
  Mux/1 -> a-cal/1, b-cal/1, c-cal/1
  a-cal/1 -> a/1
  b-cal/1 -> b/1
  c-cal/1 -> c/1

== system problematique2/Async Motor/Inverse trans1/dq2line voltage/dq2albe ==
  d : Inport
  q : Inport  Port=2
  theta : Inport  Port=3
  Mux : Mux  Inputs=3
  al-cal : Fcn  Expr=cos(u(3))*u(1) - sin(u(3))*u(2)
  be-cal : Fcn  Expr=sin(u(3))*u(1) + cos(u(3))*u(2)
  alpha : Outport  VectorParamsAs1DForOutWhenUnconnected=off
  beta : Outport  Port=2  VectorParamsAs1DForOutWhenUnconnected=off
  wires:
  Mux/1 -> al-cal/1, be-cal/1
  d/1 -> Mux/1
  al-cal/1 -> alpha/1
  q/1 -> Mux/2
  be-cal/1 -> beta/1
  theta/1 -> Mux/3

== system problematique2/Async Motor/Trans/current line2dq/abc2albe ==
  a : Inport
  b : Inport  Port=2
  c : Inport  Port=3
  Mux : Mux  Inputs=3
  al-cal : Fcn  Expr=(2/3)*u(1) - (1/3)*u(2) - (1/3)*u(3)
  q-cal : Fcn  Expr=0*u(1) + (1/sqrt(3))*(u(2) - u(3))
  alpha : Outport  VectorParamsAs1DForOutWhenUnconnected=off
  beta : Outport  Port=2  VectorParamsAs1DForOutWhenUnconnected=off
  wires:
  q-cal/1 -> beta/1
  al-cal/1 -> alpha/1
  Mux/1 -> q-cal/1, al-cal/1
  c/1 -> Mux/3
  b/1 -> Mux/2
  a/1 -> Mux/1

== system problematique2/Async Motor/Trans/current line2dq/albe2dq ==
  alpha : Inport
  beta : Inport  Port=2
  theta : Inport  Port=3
  Mux : Mux  Inputs=3
  d-cal : Fcn  Expr=cos(u(3))*u(1) + sin(u(3))*u(2)
  q-cal : Fcn  Expr=-sin(u(3))*u(1) + cos(u(3))*u(2)
  d : Outport  VectorParamsAs1DForOutWhenUnconnected=off
  q : Outport  Port=2  VectorParamsAs1DForOutWhenUnconnected=off
  wires:
  q-cal/1 -> q/1
  d-cal/1 -> d/1
  Mux/1 -> q-cal/1, d-cal/1
  theta/1 -> Mux/3
  beta/1 -> Mux/2
  alpha/1 -> Mux/1

== system problematique2/Async Motor/Transformation1/dq2line current/albe2abc ==
  alpha : Inport
  beta : Inport  Port=2
  Mux : Mux  Inputs=2
  a-cal : Fcn  Expr=u(1)
  b-cal : Fcn  Expr=(-u(1) + sqrt(3)*u(2))/2
  c-cal : Fcn  Expr=(-u(1) - sqrt(3)*u(2))/2
  a : Outport  VectorParamsAs1DForOutWhenUnconnected=off
  b : Outport  Port=2  VectorParamsAs1DForOutWhenUnconnected=off
  c : Outport  Port=3  VectorParamsAs1DForOutWhenUnconnected=off
  wires:
  alpha/1 -> Mux/1
  beta/1 -> Mux/2
  Mux/1 -> b-cal/1, c-cal/1, a-cal/1
  a-cal/1 -> a/1
  b-cal/1 -> b/1
  c-cal/1 -> c/1

== system problematique2/Async Motor/Transformation1/dq2line current/dq2albe ==
  d : Inport
  q : Inport  Port=2
  theta : Inport  Port=3
  Mux : Mux  Inputs=3
  al-cal : Fcn  Expr=cos(u(3))*u(1) - sin(u(3))*u(2)
  be-cal : Fcn  Expr=sin(u(3))*u(1) + cos(u(3))*u(2)
  alpha : Outport  VectorParamsAs1DForOutWhenUnconnected=off
  beta : Outport  Port=2  VectorParamsAs1DForOutWhenUnconnected=off
  wires:
  Mux/1 -> al-cal/1, be-cal/1
  d/1 -> Mux/1
  al-cal/1 -> alpha/1
  q/1 -> Mux/2
  be-cal/1 -> beta/1
  theta/1 -> Mux/3

== system problematique2/Async Motor/Transformation1/line2dq voltage/abc2albe ==
  a : Inport
  b : Inport  Port=2
  c : Inport  Port=3
  Mux : Mux  Inputs=3
  al-cal : Fcn  Expr=(2/3)*u(1) - (1/3)*u(2) - (1/3)*u(3)
  q-cal : Fcn  Expr=0*u(1) + (1/sqrt(3))*(u(2) - u(3))
  alpha : Outport  VectorParamsAs1DForOutWhenUnconnected=off
  beta : Outport  Port=2  VectorParamsAs1DForOutWhenUnconnected=off
  wires:
  q-cal/1 -> beta/1
  al-cal/1 -> alpha/1
  Mux/1 -> q-cal/1, al-cal/1
  c/1 -> Mux/3
  b/1 -> Mux/2
  a/1 -> Mux/1

== system problematique2/Async Motor/Transformation1/line2dq voltage/albe2dq ==
  alpha : Inport
  beta : Inport  Port=2
  theta : Inport  Port=3
  Mux : Mux  Inputs=3
  d-cal : Fcn  Expr=cos(u(3))*u(1) + sin(u(3))*u(2)
  q-cal : Fcn  Expr=-sin(u(3))*u(1) + cos(u(3))*u(2)
  d : Outport  VectorParamsAs1DForOutWhenUnconnected=off
  q : Outport  Port=2  VectorParamsAs1DForOutWhenUnconnected=off
  wires:
  q-cal/1 -> q/1
  d-cal/1 -> d/1
  Mux/1 -> q-cal/1, d-cal/1
  theta/1 -> Mux/3
  beta/1 -> Mux/2
  alpha/1 -> Mux/1
